simulink model "Res_3"  (R2018b)
settings: Solver=VariableStepAuto  StartTime=0.0  StopTime=2  RelTol=1e-3
settings Model: Creator=makha  LastModifiedBy=makha

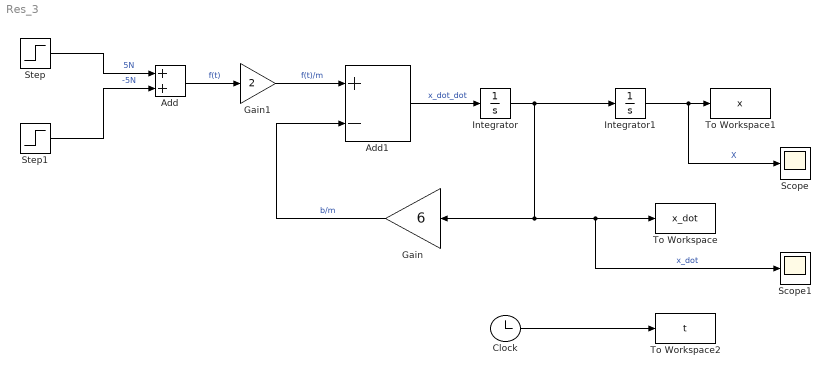
== system Res_3 ==
  Add : Sum
  Add1 : Sum  Inputs=+-
  Clock : Clock
  Gain : Gain  Gain=6
  Gain1 : Gain  Gain=2
  Integrator : Integrator
  Integrator1 : Integrator
  Scope : Scope
  Scope1 : Scope
  Step : Step  Time=0  After=5  SampleTime=0.0001
  Step1 : Step  Time=0.02  After=-5  SampleTime=0.0001
  To Workspace : ToWorkspace  VariableName=x_dot  SampleTime=-1
  To Workspace1 : ToWorkspace  VariableName=x  SampleTime=-1
  To Workspace2 : ToWorkspace  VariableName=t  SampleTime=-1
  wires:
  Step/1 -> Add/1  "5N"
  Step1/1 -> Add/2  "-5N"
  Gain/1 -> Add1/2  "b/m"
  Add1/1 -> Integrator/1  "x_dot_dot"
  Integrator/1 -> Gain/1, Scope1/1, To Workspace/1, Integrator1/1  "x_dot"
  Integrator1/1 -> Scope/1, To Workspace1/1  "X"
  Clock/1 -> To Workspace2/1
  Add/1 -> Gain1/1  "f(t)"
  Gain1/1 -> Add1/1  "f(t)/m"
